simulink library "Prop_Alpha"  (R2013b)
settings: Solver=ode45  StartTime=0.0  StopTime=10.0  RelTol=1e-3
undefined symbols (not defined in the file or in its folder): Prop
libraries: simulink x2
settings Model: Creator=mbrauer  LastModifiedBy=mbrauer

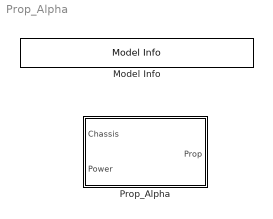
== system Prop_Alpha ==
  Model Info : simulink/Model-Wide Utilities/Model Info  InitialBlockCM=None  BlockCM=None  Frame=on  DisplayStringWithTags=Copyright 2013-2014 The MathWorks, Inc.  HorizontalTextAlignment=Center  LeftAlignmentValue=0.5  SourceBlockDiagram=Prop_Alpha  TagMaxNumber=20
  Prop_Alpha : Subsystem

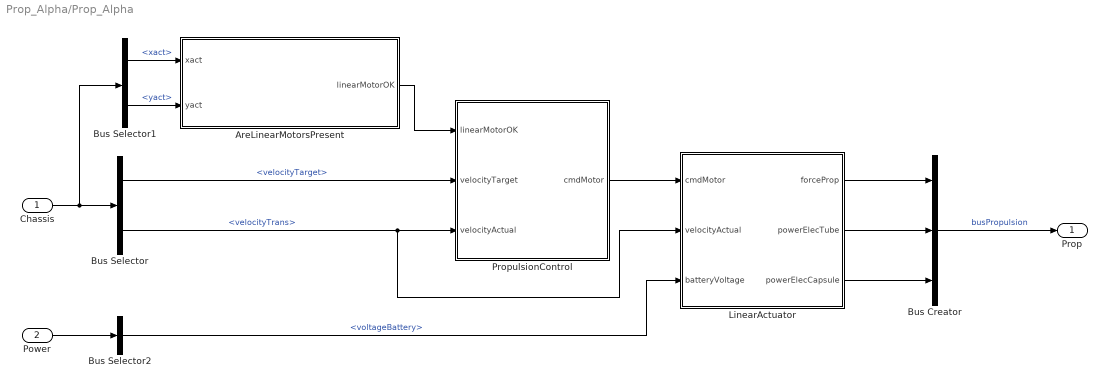
== system Prop_Alpha/Prop_Alpha ==
  Chassis : Inport
  Power : Inport  Port=2
  AreLinearMotorsPresent : Subsystem
  Bus Creator : BusCreator  Inputs=3  NonVirtualBus=on
  Bus Selector : BusSelector  OutputSignals=velocityTarget,velocityTrans
  Bus Selector1 : BusSelector  OutputSignals=GlobalFrame.xact,GlobalFrame.yact
  Bus Selector2 : BusSelector  OutputSignals=voltageBattery
  LinearActuator : Subsystem
  PropulsionControl : Subsystem
  Prop : Outport
  wires:
  AreLinearMotorsPresent/1(linearMotorOK) -> PropulsionControl/1(linearMotorOK)
  Bus Selector1/2 -> AreLinearMotorsPresent/2(yact)  "<yact>"
  Bus Selector1/1 -> AreLinearMotorsPresent/1(xact)  "<xact>"
  Power/1 -> Bus Selector2/1
  Bus Selector2/1 -> LinearActuator/3(batteryVoltage)  "<voltageBattery>"
  LinearActuator/1(forceProp) -> Bus Creator/1
  Bus Selector/1 -> PropulsionControl/2(velocityTarget)  "<velocityTarget>"
  Bus Selector/2 -> LinearActuator/2(velocityActual), PropulsionControl/3(velocityActual)  "<velocityTrans>"
  Chassis/1 -> Bus Selector/1, Bus Selector1/1
  LinearActuator/3(powerElecCapsule) -> Bus Creator/3
  LinearActuator/2(powerElecTube) -> Bus Creator/2
  Bus Creator/1 -> Prop/1  "busPropulsion"
  PropulsionControl/1(cmdMotor) -> LinearActuator/1(cmdMotor)

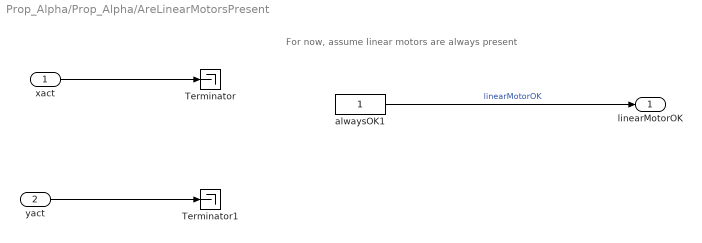
== system Prop_Alpha/Prop_Alpha/AreLinearMotorsPresent ==
  note: For now, assume linear motors are always present
  xact : Inport
  yact : Inport  Port=2
  Terminator : Terminator
  Terminator1 : Terminator
  alwaysOK1 : Constant
  linearMotorOK : Outport
  wires:
  alwaysOK1/1 -> linearMotorOK/1  "linearMotorOK"
  xact/1 -> Terminator/1
  yact/1 -> Terminator1/1

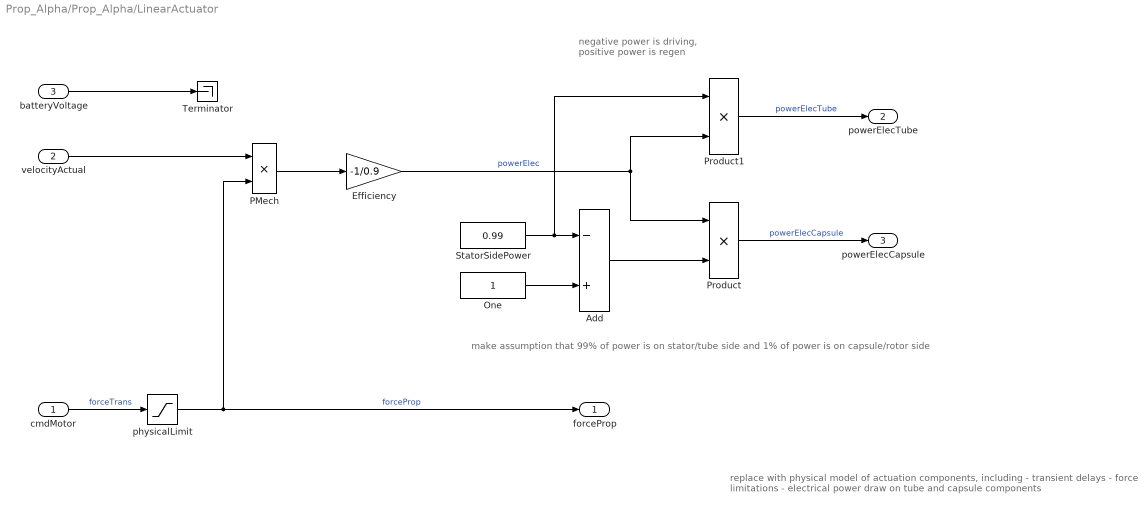
== system Prop_Alpha/Prop_Alpha/LinearActuator ==
  note: negative power is driving,
      | positive power is regen
  note: make assumption that 99% of power is on stator/tube side and 1% of power is on capsule/rotor side
  note: replace with physical model of actuation components, including
      | - transient delays
      | - force limitations
      | - electrical power draw on tube and capsule components
  cmdMotor : Inport
  velocityActual : Inport  Port=2
  batteryVoltage : Inport  Port=3
  Add : Sum  Inputs=-+
  Efficiency : Gain  Gain=-1/0.9
  One : Constant
  PMech : Product  Inputs=**
  Product : Product
  Product1 : Product
  StatorSidePower : Constant  Value=0.99
  Terminator : Terminator
  physicalLimit : Saturate  UpperLimit=Prop.MaxForce  LowerLimit=-Prop.MaxForce
  forceProp : Outport
  powerElecTube : Outport  Port=2
  powerElecCapsule : Outport  Port=3
  wires:
  cmdMotor/1 -> physicalLimit/1  "forceTrans"
  Product1/1 -> powerElecTube/1  "powerElecTube"
  Product/1 -> powerElecCapsule/1  "powerElecCapsule"
  batteryVoltage/1 -> Terminator/1
  physicalLimit/1 -> forceProp/1, PMech/2  "forceProp"
  velocityActual/1 -> PMech/1
  PMech/1 -> Efficiency/1
  Efficiency/1 -> Product1/2, Product/1  "powerElec"
  One/1 -> Add/2
  StatorSidePower/1 -> Product1/1, Add/1
  Add/1 -> Product/2

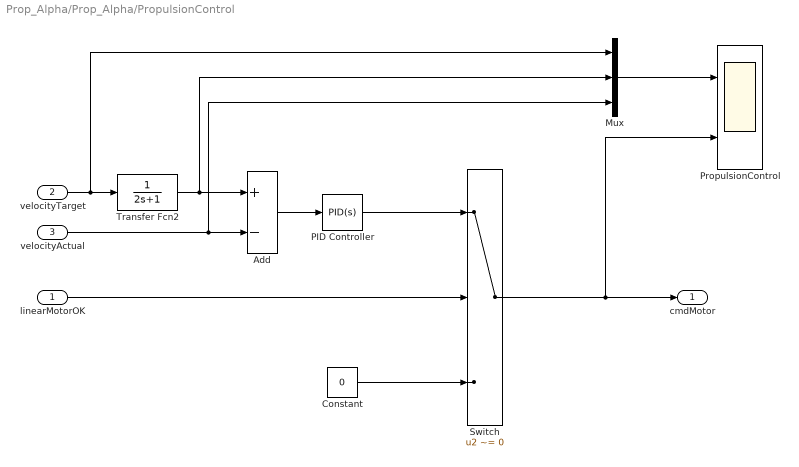
== system Prop_Alpha/Prop_Alpha/PropulsionControl ==
  linearMotorOK : Inport
  velocityTarget : Inport  Port=2
  velocityActual : Inport  Port=3
  Add : Sum  Inputs=+-
  Constant : Constant  Value=0
  Mux : Mux  Inputs=3
  PID Controller : simulink/Continuous/PID Controller  Controller=PID  TimeDomain=Continuous-time  SampleTime=1  IntegratorMethod=Forward Euler  FilterMethod=Forward Euler  Form=Parallel  P=3500  I=500  D=500  N=0.1  InitialConditionSource=internal  InitialConditionForIntegrator=0  InitialConditionForFilter=0  ExternalReset=none  LimitOutput=on  UpperSaturationLimit=Prop.MaxForce  LowerSaturationLimit=-Prop.MaxForce  LinearizeAsGain=on  AntiWindupMode=back-calculation  Kb=1  TrackingMode=off  Kt=1  PParamMin=[]  PParamMax=[]  IParamMin=[]  IParamMax=[]  DParamMin=[]  DParamMax=[]  NParamMin=[]  NParamMax=[]  KbParamMin=[]  KbParamMax=[]  KtParamMin=[]  KtParamMax=[]  POutMin=[]  POutMax=[]  IOutMin=[]  IOutMax=[]  DOutMin=[]  DOutMax=[]  NOutMin=[]  NOutMax=[]  KbOutMin=[]  KbOutMax=[]  KtOutMin=[]  KtOutMax=[]  IntegratorOutMin=[]  IntegratorOutMax=[]  FilterOutMin=[]  FilterOutMax=[]  SumOutMin=[]  SumOutMax=[]  SumI1OutMin=[]  SumI1OutMax=[]  SumI2OutMin=[]  SumI2OutMax=[]  SumI3OutMin=[]  SumI3OutMax=[]  SumDOutMin=[]  SumDOutMax=[]  SaturationOutMin=[]  SaturationOutMax=[]  IntegratorContinuousStateAttributes=''  IntegratorStateMustResolveToSignalObject=off  IntegratorRTWStateStorageClass=Auto  FilterContinuousStateAttributes=''  FilterStateMustResolveToSignalObject=off  FilterRTWStateStorageClass=Auto
  PropulsionControl : Scope  NumInputPorts=2
      settings: TimeRange=250  YMin=130~-15000  YMax=270~85000  SaveName=ScopeData2  MaxDataPoints=500000  Decimation=10
  Switch : Switch  Criteria=u2 ~= 0
  Transfer Fcn2 : TransferFcn  Denominator=[2 1]
  cmdMotor : Outport
  wires:
  PID Controller/1 -> Switch/1
  velocityActual/1 -> Mux/3, Add/2
  velocityTarget/1 -> Mux/1, Transfer Fcn2/1
  linearMotorOK/1 -> Switch/2
  Constant/1 -> Switch/3
  Add/1 -> PID Controller/1
  Switch/1 -> PropulsionControl/2, cmdMotor/1
  Mux/1 -> PropulsionControl/1
  Transfer Fcn2/1 -> Mux/2, Add/1
